simulink model "AHRS_voter_Harness_triple_sensor"  (R2019b)
settings: Solver=FixedStepDiscrete  StartTime=0.0  StopTime=10.0  FixedStep=0.01  RelTol=1e-3  EnableMultiTasking=on
settings Model: DataDictionary=HeliSystemDD.sldd  Creator=bpotter  LastModifiedBy=bpotter
settings DataIOCC: LimitDataPoints=on  SaveFormat=Array  ReturnWorkspaceOutputs=off
settings OptimizationCC: BlockReduction=off  ConditionallyExecuteInputs=off  DefaultParameterBehavior=Inlined  UseDivisionForNetSlopeComputation=on  InitFltsAndDblsToZero=on  EfficientFloat2IntCast=on  EfficientMapNaN2IntZero=off  LifeSpan=inf  MaxStackSize=inf  EfficientTunableParamExpr=on
settings DebuggingCC: SignalInfNanChecking=error  SignalRangeChecking=error  ReadBeforeWriteMsg=EnableAllAsError  WriteAfterWriteMsg=EnableAllAsError  WriteAfterReadMsg=EnableAllAsError  AlgebraicLoopMsg=error  ArtificialAlgebraicLoopMsg=error  SaveWithDisabledLinksMsg=error  SaveWithParameterizedLinksMsg=error  BlockPriorityViolationMsg=error  SolverPrmCheckMsg=error  InheritedTsInSrcMsg=error  SingleTaskRateTransMsg=error  TasksWithSamePriorityMsg=error  SigSpecEnsureSampleTimeMsg=error  CheckMatrixSingularityMsg=error  IntegerOverflowMsg=error  ParameterUnderflowMsg=error  ParameterPrecisionLossMsg=error  ParameterTunabilityLossMsg=error  UnderSpecifiedDataTypeMsg=error  UnnecessaryDatatypeConvMsg=warning  VectorMatrixConversionMsg=error  SignalLabelMismatchMsg=error  UnconnectedInputMsg=error  UnconnectedOutputMsg=error  UnconnectedLineMsg=error  SFcnCompatibilityMsg=error  UniqueDataStoreMsg=error  BusObjectLabelMismatch=error  RootOutportRequireBusObject=error  AssertControl=DisableAll  AllowSymbolicDim=off  ModelReferenceIOMsg=error  ModelReferenceIOMismatchMessage=error  UnknownTsInhSupMsg=error  ModelReferenceDataLoggingMessage=error  StateNameClashWarn=warning  PregeneratedLibrarySubsystemCodeDiagnostic=none  StrictBusMsg=ErrorOnBusTreatedAsVector  NonBusSignalsTreatedAsBus=error  SFInvalidInputDataAccessInChartInitDiag=error  SFTransitionOutsideNaturalParentDiag=error  SFUnreachableExecutionPathDiag=error  SFUndirectedBroadcastEventsDiag=error  SFTransitionActionBeforeConditionDiag=error  SFExecutionAtInitializationDiag=none  IntegerSaturationMsg=error  ArithmeticOperatorsInVariantConditions=warning
settings HardwareCC: ProdBitPerPointer=32  ProdBitPerSizeT=32  ProdBitPerPtrDiffT=32  ProdWordSize=32  ProdHWDeviceType=Intel->x86-32 (Windows32)  TargetIntDivRoundTo=Zero
settings ModelReferenceCC: PropagateSignalLabelsOutOfModel=off
settings SFSimCC: SimUseLocalCustomCode=off  CompileTimeRecursionLimit=0  EnableRuntimeRecursion=off  MATLABDynamicMemAlloc=off  CustomCodeUndefinedFunction=UseInterfaceOnly
settings RTWCC: SystemTargetFile=ert.tlc  TemplateMakefile=ert_default_tmf  GenerateReport=on  RTWUseLocalCustomCode=off  IncludeHyperlinkInReport=on  LaunchReport=on  PortableWordSizes=on  GenerateTraceInfo=on  GenerateTraceReport=on  GenerateTraceReportSl=on  GenerateTraceReportSf=on  GenerateTraceReportEml=on
settings CodeAppCC: ForceParamTrailComments=on  IgnoreCustomStorageClasses=off  MangleLength=4  StateflowObjectComments=on  ReqsInCode=on
settings ERTTargetCC: TargetLangStandard=C99 (ISO)  UtilityFuncGeneration=Shared location  MultiwordLength=2048  GenerateSampleERTMain=on  IncludeMdlTerminateFcn=off  SuppressErrorStatus=on  SupportAbsoluteTime=off  SupportNonFinite=off  ParenthesesLevel=Maximum  CastingMode=Standards  GenerateSharedConstants=off  ERTCustomFileTemplate=example_file_process.tlc  ERTFilePackagingFormat=Compact  PreserveExpressionOrder=on  PreserveIfCondition=on  ConvertIfToSwitch=off  SuppressUnreachableDefaultCases=off  EnableSignedLeftShifts=off  EnableSignedRightShifts=off
settings ConfigComp: CovEnable=on  CovScope=ReferencedModels  CovIncludeTopModel=off  CovMetricSettings=dcmtrzoibe  CovHTMLOptions=-sRT=1 -sVT=0 -aTS=1 -bRG=1 -bTC=1 -hTR=1 -nFC=0 -scm=1 -bcm=1 -xEv=0  CovSaveCumulativeToWorkspaceVar=on  CovCumulativeVarName=AHRScovCumData  CovCumulativeReport=on  CovModelRefEnable=on  CovExternalEMLEnable=off  CovSFcnEnable=off  PSVerificationMode=BugFinder  PSResultDir=\BugFinder_results  PSModelRefVerifDepth=All  PSAutoStubLUT=off  DVMakeOutputFilesUnique=off  DVModelCoverageObjectives=MCDC  DVTestSuiteOptimization=IndividualObjectives  DVIgnoreCovSatisfied=on  DVCoverageDataFile=simulation_results\AHRS_voter_cov.cvt  DVIncludeRelationalBoundary=on  DVSaveDataFile=off  DVSaveReport=on  DVReportPDFFormat=on  DVRebuildModelRepresentation=Always

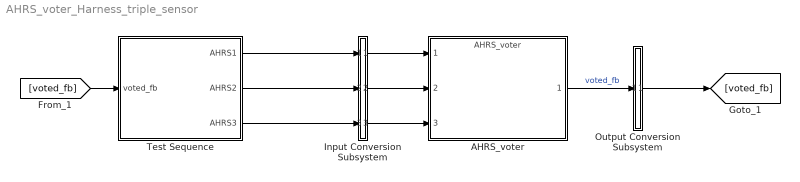
== system AHRS_voter_Harness_triple_sensor ==
  AHRS_voter : ModelReference  ModelNameDialog=AHRS_voter  SimulationMode=Normal  ModelReferenceVersion=1.66
  Input Conversion Subsystem : Subsystem  Tag=__SLT_ICS__  Description=|
      | Signal spec.
      | and routing
      settings: AttributesFormatString=%<Description>
  Output Conversion Subsystem : Subsystem  Tag=__SLT_OCS__  Description=|
      | Signal spec.
      | and routing
      settings: AttributesFormatString=%<Description>
  Test Sequence : Test Sequence  TreatAsAtomicUnit=on
  wires:
  Test Sequence/1(AHRS1) -> Input Conversion Subsystem/1(Inport_1)
  Test Sequence/2(AHRS2) -> Input Conversion Subsystem/2(Inport_2)
  Test Sequence/3(AHRS3) -> Input Conversion Subsystem/3(Inport_3)
  [voted_fb] -> Test Sequence/1(voted_fb)
  Output Conversion Subsystem/1(Outport_1) -> [voted_fb]
  Input Conversion Subsystem/1(Outport_1) -> AHRS_voter/1
  Input Conversion Subsystem/2(Outport_2) -> AHRS_voter/2
  Input Conversion Subsystem/3(Outport_3) -> AHRS_voter/3
  AHRS_voter/1 -> Output Conversion Subsystem/1(Inport_1)  "voted_fb"

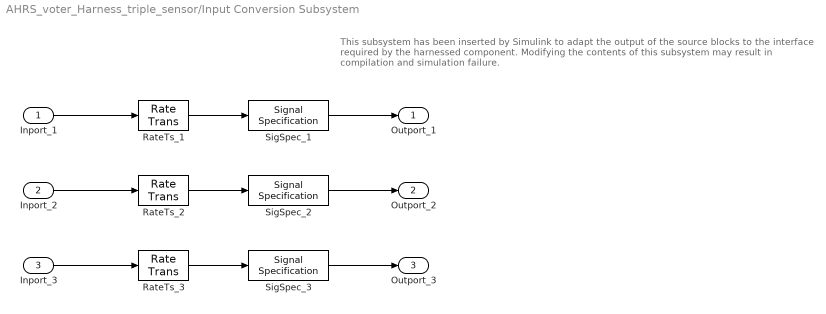
== system AHRS_voter_Harness_triple_sensor/Input Conversion Subsystem ==
  note: This subsystem has been inserted by Simulink to adapt the output of the source blocks to the interface required by the harnessed component.
      |  Modifying the contents of this subsystem may result in compilation and simulation failure.
  Inport_1 : Inport
  Inport_2 : Inport  Port=2
  Inport_3 : Inport  Port=3
  RateTs_1 : RateTransition  OutPortSampleTime=0.01
  RateTs_2 : RateTransition  OutPortSampleTime=0.01
  RateTs_3 : RateTransition  OutPortSampleTime=0.01
  SigSpec_1 : SignalSpecification  OutDataTypeStr=Bus: AHRS_Bus  Dimensions=[1]  SampleTime=0.01  BusOutputAsStruct=on
  SigSpec_2 : SignalSpecification  OutDataTypeStr=Bus: AHRS_Bus  Dimensions=[1]  SampleTime=0.01  BusOutputAsStruct=on
  SigSpec_3 : SignalSpecification  OutDataTypeStr=Bus: AHRS_Bus  Dimensions=[1]  SampleTime=0.01  BusOutputAsStruct=on
  Outport_1 : Outport  VectorParamsAs1DForOutWhenUnconnected=off
  Outport_2 : Outport  Port=2  VectorParamsAs1DForOutWhenUnconnected=off
  Outport_3 : Outport  Port=3  VectorParamsAs1DForOutWhenUnconnected=off
  wires:
  SigSpec_1/1 -> Outport_1/1
  RateTs_1/1 -> SigSpec_1/1
  Inport_1/1 -> RateTs_1/1
  SigSpec_2/1 -> Outport_2/1
  RateTs_2/1 -> SigSpec_2/1
  Inport_2/1 -> RateTs_2/1
  SigSpec_3/1 -> Outport_3/1
  RateTs_3/1 -> SigSpec_3/1
  Inport_3/1 -> RateTs_3/1

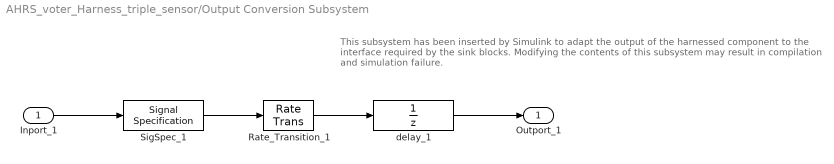
== system AHRS_voter_Harness_triple_sensor/Output Conversion Subsystem ==
  note: This subsystem has been inserted by Simulink to adapt the output of the harnessed component to the interface required by the sink blocks.
      |  Modifying the contents of this subsystem may result in compilation and simulation failure.
  Inport_1 : Inport
  Rate_Transition_1 : RateTransition  OutPortSampleTimeOpt=Inherit
  SigSpec_1 : SignalSpecification  OutDataTypeStr=double  Dimensions=[5]  SampleTime=0.01
  delay_1 : UnitDelay  SampleTime=-1
  Outport_1 : Outport  VectorParamsAs1DForOutWhenUnconnected=off
  wires:
  Inport_1/1 -> SigSpec_1/1
  SigSpec_1/1 -> Rate_Transition_1/1
  Rate_Transition_1/1 -> delay_1/1
  delay_1/1 -> Outport_1/1

== stateflow chart AHRS_voter_Harness_triple_sensor/Test Sequence ==
  settings: stateMachineType=SIMPLIFIED_MACHINE
  state Run
    %% Initialize data outputs.
    AHRS1.theta = 0;
    AHRS1.phi = 0;
    AHRS1.psi = 0;
    AHRS1.r = 0;
    AHRS1.q = 0;
    AHRS1.p = 0;
    AHRS1.valid = true;
    AHRS2.theta = 0;
    AHRS2.phi = 0;
    AHRS2.psi = 0;
    AHRS2.r = 0;
    AHRS2.q = 0;
    AHRS2.p = 0;
    AHRS2.valid = true;
    AHRS3.theta = 0;
    AHRS3.phi = 0;
    AHRS3.psi = 0;
    AHRS3.r = 0;
    AHRS3.q = 0;
    AHRS3.p = 0;
    AHRS3.valid = true;
  state step_1
    % Test that all outputs are set to zero uisng the tolerance
    verify(abs(voted_fb(1))<Tol, 'Zero output condition failed for theta');
    verify(abs(voted_fb(2))<Tol, 'Zero output condition failed for phi');
    verify(abs(voted_fb(3))<Tol, 'Zero output condition failed for r');
    verify(abs(voted_fb(4))<Tol, 'Zero output condition failed for q');
    verify(abs(voted_fb(5))<Tol, 'Zero output condition failed for p');
  state step_2
    % Set data to different values for each AHRS and each element
    AHRS1.theta = 1;
    AHRS1.phi = -2;
    AHRS1.psi = 0;
    AHRS1.r = 3;
    AHRS1.q = 4;
    AHRS1.p = 0;
    AHRS2.theta = -1;
    AHRS2.phi = 2;
    AHRS2.psi = 0;
    AHRS2.r = -3;
    AHRS2.q = -4;
    AHRS2.p = -5;
    AHRS3.theta = 5;
    AHRS3.phi = 4;
    AHRS3.psi = 0;
    AHRS3.r = 3;
    AHRS3.q = -2;
    AHRS3.p = 1;
  state step_3
    % Test that each element is the mid value, based on the three inputs
    verify((voted_fb(1)-AHRS1.theta)<Tol, 'Mid value selection failed for AHRS1 theta');
    verify((voted_fb(2)-AHRS2.phi)<Tol, 'Mid value selection failed for AHRS2 phi');
    verify((voted_fb(3)-AHRS3.r)<Tol, 'Mid value selection failed for AHRS3 r');
    verify((voted_fb(4)-AHRS3.q)<Tol, 'Mid value selection failed for AHRS3 q');
    verify((voted_fb(5)-AHRS1.p)<Tol, 'Mid value selection failed for AHRS1 p');
  state step_4
    % Set data to different vlaues at or near full positive range for each AHRS and each element
    AHRS1.theta = 180;
    AHRS1.phi = 179;
    AHRS1.psi = 0;
    AHRS1.r = 180;
    AHRS1.q = 178;
    AHRS1.p = 178;
    AHRS2.theta = 179;
    AHRS2.phi = 180;
    AHRS2.psi = 0;
    AHRS2.r = 179;
    AHRS2.q = 179;
    AHRS2.p = 180;
    AHRS3.theta = 178;
    AHRS3.phi = 178;
    AHRS3.psi = 0;
    AHRS3.r = 178;
    AHRS3.q = 180;
    AHRS3.p = 179;
  state step_5
    % Test that each element is the mid value, based on the three inputs
    verify((voted_fb(1)-AHRS2.theta)<Tol, 'Mid value selection failed for AHRS2 theta');
    verify((voted_fb(2)-AHRS1.phi)<Tol, 'Mid value selection failed for AHRS1 phi');
    verify((voted_fb(3)-AHRS2.r)<Tol, 'Mid value selection failed for AHRS2 r');
    verify((voted_fb(4)-AHRS2.q)<Tol, 'Mid value selection failed for AHRS2 q');
    verify((voted_fb(5)-AHRS3.p)<Tol, 'Mid value selection failed for AHRS3 p');
  state step_6
    % Set data to different vlaues at or near full negative range for each AHRS and each element
    AHRS1.theta = -180;
    AHRS1.phi = -178;
    AHRS1.psi = 0;
    AHRS1.r = -179;
    AHRS1.q = -179;
    AHRS1.p = -180;
    AHRS2.theta = -178;
    AHRS2.phi = -180;
    AHRS2.psi = 0;
    AHRS2.r = -180;
    AHRS2.q = -178;
    AHRS2.p = -179;
    AHRS3.theta = -179;
    AHRS3.phi = -179;
    AHRS3.psi = 0;
    AHRS3.r = -178;
    AHRS3.q = -180;
    AHRS3.p = -178;
  state step_7
    % Test that each element is the mid value, based on the three inputs
    verify((voted_fb(1)-AHRS3.theta)<Tol, 'Mid value selection failed for AHRS3 theta');
    verify((voted_fb(2)-AHRS3.phi)<Tol, 'Mid value selection failed for AHRS3 phi');
    verify((voted_fb(3)-AHRS1.r)<Tol, 'Mid value selection failed for AHRS1 r');
    verify((voted_fb(4)-AHRS1.q)<Tol, 'Mid value selection failed for AHRS1 q');
    verify((voted_fb(5)-AHRS2.p)<Tol, 'Mid value selection failed for AHRS2 p');
  (default) -> Run
  Run -> step_1 : [
      | after(1, sec)
      | ]
  step_1 -> step_2 : [
      | true
      | ]
  step_2 -> step_3 : [
      | after(1, sec)
      | ]
  step_3 -> step_4 : [
      | true
      | ]
  step_4 -> step_5 : [
      | after(1, sec)
      | ]
  step_5 -> step_6 : [
      | true
      | ]
  step_6 -> step_7 : [
      | after(1, sec)
      | ]
  data: voted_fb input double size=[5]; AHRS1 output Bus: AHRS_Bus size=[1]; AHRS2 output Bus: AHRS_Bus size=[1]; AHRS3 output Bus: AHRS_Bus size=[1]; Tol local =1e-7
